simulink model "photorealisticSimulationEngi"  (R2021b)
settings: Solver=FixedStepAuto  StartTime=0.0  StopTime=50  RelTol=1e-3  EnableMultiTasking=on
undefined symbols (not defined in the file): Earth, initialConditions, Lidar, lidarAngles, UAV, UAVSampleTime, uavScenarioBlock, WGS84
libraries: uavsimlib x5, robotcorelib x3, simulink x3, uavutilslib x1, mspfiltlib x1, sim3dcameralib x1, sensorgpslib x1, mspsensorlib x1, aerolibtransform2 x1, sim3dphyssensorlib x1, sim3dlib x1, uavsim3dlib x1
settings Model: DataDictionary=uavPackageDeliveryDataDict.sldd  ModifiedByFormat=The MathWorks, Inc.  Creator=The MathWorks, Inc.  LastModifiedBy=The MathWorks, Inc.
settings SolverCC: AlgebraicLoopSolver=TrustRegion  AutoInsertRateTranBlk=on
settings DataIOCC: LimitDataPoints=on  SaveOutput=off  SaveTime=off  ReturnWorkspaceOutputs=off
settings OptimizationCC: EnhancedBackFolding=on  PassReuseOutputArgsThreshold=0  ZeroExternalMemoryAtStartup=off  ZeroInternalMemoryAtStartup=off  MaxStackSize=64  OptimizeBlockOrder=speed  DifferentSizesBufferReuse=on  OptimizationCustomize=off
settings DebuggingCC: ParameterPrecisionLossMsg=none  ParameterTunabilityLossMsg=error  AllowSymbolicDim=off  SFUnexpectedBacktrackingDiag=warning  SFNoUnconditionalDefaultTransitionDiag=warning  SFExecutionAtInitializationDiag=none  SFMachineParentedDataDiag=warning  ArithmeticOperatorsInVariantConditions=warning
settings HardwareCC: ProdBitPerPointer=32  ProdBitPerSizeT=32  ProdBitPerPtrDiffT=32  ProdLargestAtomicFloat=None  ProdIntDivRoundTo=Undefined  ProdEndianess=Unspecified  ProdWordSize=32  ProdHWDeviceType=Generic->Unspecified (assume 32-bit Generic)
settings ModelReferenceCC: ModelReferenceNumInstancesAllowed=Single  PropagateSignalLabelsOutOfModel=off
settings SFSimCC: SimUseLocalCustomCode=off  MATLABDynamicMemAlloc=off  CustomCodeUndefinedFunction=UseInterfaceOnly  SimTargetLang=C++
settings RTWCC: GenerateReport=on  RTWUseLocalCustomCode=off  LaunchReport=on  TargetLang=C++
settings CodeAppCC: ForceParamTrailComments=on  OperatorAnnotations=on
settings GRTTargetCC: TargetLangStandard=C89/C90 (ANSI)  CodeInterfacePackaging=C++ class
settings ConfigComp: CovMetricSettings=dw  CovSaveCumulativeToWorkspaceVar=on  CovSaveSingleToWorkspaceVar=on  CovExternalEMLEnable=off

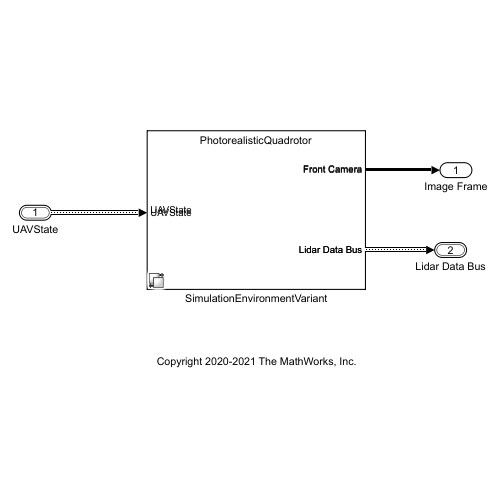
[thumbnail: Simulink's stored preview of the top-level diagram]
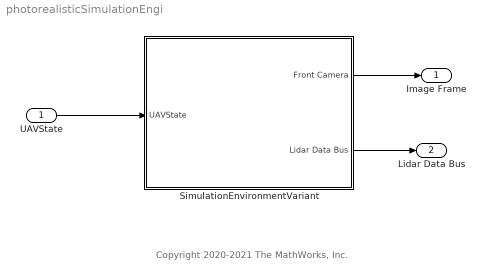
== system photorealisticSimulationEngi ==
  note: Copyright 2020-2021 The MathWorks, Inc.
  UAVState : Inport  OutDataTypeStr=Bus: uavStateBus  BusOutputAsStruct=on
  SimulationEnvironmentVariant : Subsystem  Variant=on  PropagateVariantConditions=on
  Image Frame : Outport
  Lidar Data Bus : Outport  Port=2  OutDataTypeStr=Bus: LidarData
  wires:
  UAVState/1 -> SimulationEnvironmentVariant/1(UAVState)
  SimulationEnvironmentVariant/1(Front Camera) -> Image Frame/1
  SimulationEnvironmentVariant/2(Lidar Data Bus) -> Lidar Data Bus/1

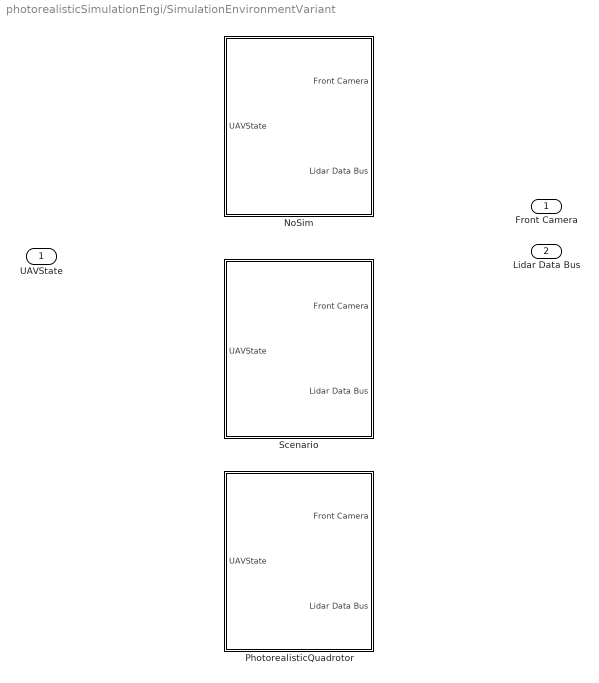
== system photorealisticSimulationEngi/SimulationEnvironmentVariant ==
  UAVState : Inport  OutDataTypeStr=Bus: uavStateBus  PortDimensions=[1 1]  BusOutputAsStruct=on
  NoSim : Subsystem  VariantControl=isPhotoRealisticSim==0
  PhotorealisticQuadrotor : Subsystem  VariantControl=isPhotoRealisticSim==2
  Scenario : Subsystem  VariantControl=isPhotoRealisticSim==1
  Front Camera : Outport  PortDimensions=[ 480 752 3]
  Lidar Data Bus : Outport  Port=2

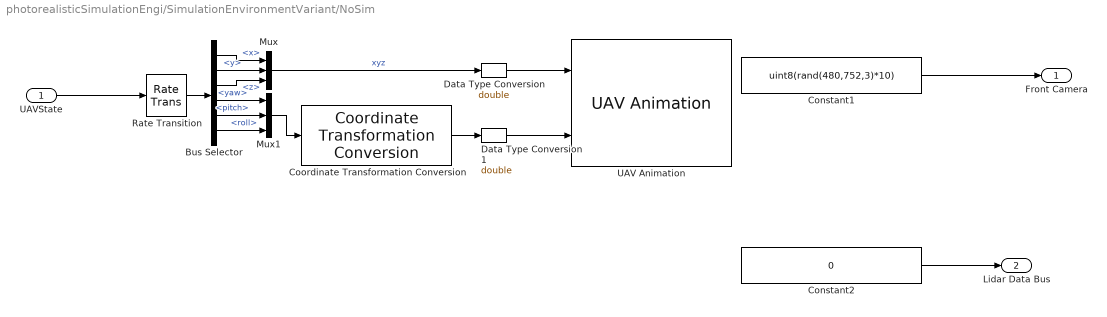
== system photorealisticSimulationEngi/SimulationEnvironmentVariant/NoSim ==
  UAVState : Inport  OutDataTypeStr=Bus: uavStateBus  PortDimensions=[1 1]  SampleTime=UAVSampleTime  BusOutputAsStruct=on
  Bus Selector : BusSelector  OutputSignals=pos_vel.x,pos_vel.y,pos_vel.z,attitude.yaw,attitude.pitch,attitude.roll
  Constant1 : Constant  Value=uint8(rand(480,752,3)*10)
  Constant2 : Constant  Value=0  OutDataTypeStr=Bus: LidarData
  Coordinate Transformation Conversion : robotcorelib/Coordinate Transformation Conversion  InputRepresentation=Euler Angles  InputEulerSequence=ZYX  ShowTrVecInputPort=on  OutputRepresentation=Quaternion  OutputEulerSequence=ZYX  ShowTrVecOutputPort=on  SimulateUsing=Code generation
  Data Type Conversion : DataTypeConversion  OutDataTypeStr=double
  Data Type Conversion1 : DataTypeConversion  OutDataTypeStr=double
  Mux : Mux  Inputs=3
  Mux1 : Mux  Inputs=3
  Rate Transition : RateTransition  OutPortSampleTime=UAVSampleTime*200
  UAV Animation : uavutilslib/UAV Animation  UAVType=Multirotor  UAVSize=1  InertialZDirection=Down  SampleTime=UAVSampleTime*200
      settings: SourceProductName=UAV Toolbox
  Front Camera : Outport  OutDataTypeStr=uint8  PortDimensions=[480 752 3]
  Lidar Data Bus : Outport  Port=2
  wires:
  Constant1/1 -> Front Camera/1
  Constant2/1 -> Lidar Data Bus/1
  Bus Selector/1 -> Mux/1  "<x>"
  Bus Selector/2 -> Mux/2  "<y>"
  Bus Selector/3 -> Mux/3  "<z>"
  Mux/1 -> Data Type Conversion/1  "xyz"
  Bus Selector/6 -> Mux1/3  "<roll>"
  Bus Selector/5 -> Mux1/2  "<pitch>"
  Bus Selector/4 -> Mux1/1  "<yaw>"
  Coordinate Transformation Conversion/1 -> Data Type Conversion1/1
  Mux1/1 -> Coordinate Transformation Conversion/1
  Data Type Conversion1/1 -> UAV Animation/2
  UAVState/1 -> Rate Transition/1
  Data Type Conversion/1 -> UAV Animation/1
  Rate Transition/1 -> Bus Selector/1

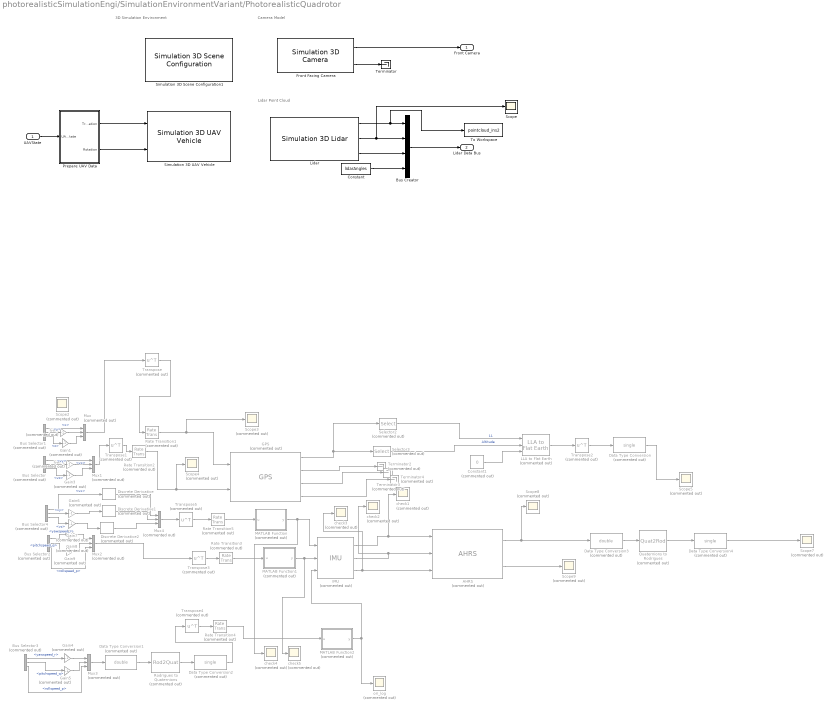
== system photorealisticSimulationEngi/SimulationEnvironmentVariant/PhotorealisticQuadrotor ==
  note: 3D Simulation Environment
  note: Camera Model
  note: Lidar Point Cloud
  UAVState : Inport  PortDimensions=[1 1]  SampleTime=[0.01,0]  BusOutputAsStruct=on
  AHRS : mspfiltlib/AHRS  Commented=on  DispRefFrame=NED  DecimationFactor=1  InitialProcessNoise=ahrsfilter.defaultProcessNoise  OrientationFormat=quaternion  SimulateUsing=Interpreted execution  AccelerometerNoise=0.0001924722  GyroscopeNoise=9.1385e-5  MagnetometerNoise=0.1  GyroscopeDriftNoise=3.0462e-13  LinearAccelerationNoise=0.0096236100000000012  MagneticDisturbanceNoise=0.5  LinearAccelerationDecayFactor=0.5  MagneticDisturbanceDecayFactor=0.5  ExpectedMagneticFieldStrength=50
      settings: SourceProductBaseCode=TF,NV
  Bus Creator : BusCreator  Inputs=4  OutDataTypeStr=Bus: LidarData  NonVirtualBus=on
      settings: InheritFromInputs=off
  Bus Selector : BusSelector  Commented=on  OutputSignals=pos_vel.vx,pos_vel.vy,pos_vel.vz
  Bus Selector1 : BusSelector  Commented=on  OutputSignals=pos_vel.x,pos_vel.y,pos_vel.z
  Bus Selector2 : BusSelector  Commented=on  OutputSignals=attitude.yawspeed_r,attitude.pitchspeed_q,attitude.rollspeed_p
  Bus Selector3 : BusSelector  Commented=on  OutputSignals=attitude.yawspeed_r,attitude.pitchspeed_q,attitude.rollspeed_p
  Bus Selector4 : BusSelector  Commented=on  OutputSignals=pos_vel.vx,pos_vel.vy,pos_vel.vz
  Constant : Constant  Value=lidarAngles
  Constant1 : Constant  Commented=on  Value=0
  Data Type Conversion : DataTypeConversion  Commented=on  OutDataTypeStr=single
  Data Type Conversion1 : DataTypeConversion  Commented=on  OutDataTypeStr=double
  Data Type Conversion2 : DataTypeConversion  Commented=on  OutDataTypeStr=single
  Data Type Conversion3 : DataTypeConversion  Commented=on  OutDataTypeStr=double
  Data Type Conversion4 : DataTypeConversion  Commented=on  OutDataTypeStr=single
  Discrete Derivative : simulink/Discrete/Discrete Derivative  Commented=on  gainval=1.0  ICPrevScaledInput=0.0  OutMin=[]  OutMax=[]  OutDataType=fixdt(1, 16)  OutScaling=2^-10  DoSatur=off
  Discrete Derivative1 : simulink/Discrete/Discrete Derivative  Commented=on  gainval=1.0  ICPrevScaledInput=0.0  OutMin=[]  OutMax=[]  OutDataType=fixdt(1, 16)  OutScaling=2^-10  DoSatur=off
  Discrete Derivative2 : simulink/Discrete/Discrete Derivative  Commented=on  gainval=1.0  ICPrevScaledInput=0.0  OutMin=[]  OutMax=[]  OutDataType=fixdt(1, 16)  OutScaling=2^-10  DoSatur=off
  Front Facing Camera : sim3dcameralib/Simulation 3D Camera  Priority=1  sensorTag=Sim3dSensor2  sensorId=2  sensorName=Sim3dSensor2  vehTagList={'Scene Origin';'SimulinkVehicle1'}  vehTag=SimulinkVehicle1  mountLoc=Origin  offsetFlag=on  tmountOffset=[0 0 -0.15]  extTmount=off  rmountOffset=[0, 0, 0]  extRmount=off  FocalLength=[1109, 1109]  OpticalCenter=[376, 240]  ImageSize=[480, 752]  RadialDistortion=[0, 0]  TangentialDistortion=[0, 0]  SensorSkew=0  DepthOutportEnabled=on  SemanticOutportEnabled=off  TransformOutportEnabled=off  SampleTime=UAVSampleTime*20  mountPoint=[0 0 -0.15]  mountOrientation=[0 0 0]  aMode=4  ID=2
      settings: SourceProductBaseCode=AE,DR,UV,VE
  GPS : sensorgpslib/GPS  Commented=on  DispRefFrame=NED  PositionInputFormat=Local  ReferenceLocation=[41.8856528 -87.6556726 0]  HorizontalPositionAccuracy=1.6  VerticalPositionAccuracy=3  VelocityAccuracy=0.1  DecayFactor=0.999  SeedDouble=67  SimulateUsing=Interpreted execution
      settings: SourceProductBaseCode=TF,NV,UV
  Gain{,1..9} (10 alike) : Gain  Commented=on  Gain=-1
  IMU : mspsensorlib/IMU  Commented=on  DispRefFrame=NED  Temperature=25  MagneticFieldNED=[ 27.5550, -2.4169, -16.0849 ]  MagneticFieldENU=[ -2.4169, 27.5550, 16.0849 ]  SeedDouble=67  SimulateUsing=Interpreted execution  AccelParamsMeasurementRange=Inf  AccelParamsResolution=0  AccelParamsConstantBias=[ 0, 0, 0 ]  AccelParamsAxesMisalignment=[ 100, 0, 0; 0, 100, 0; 0, 0, 100 ]  AccelParamsNoiseDensity=[ 0, 0, 0 ]  AccelParamsBiasInstability=[ 0, 0, 0 ]  AccelParamsRandomWalk=[ 0, 0, 0 ]  AccelParamsTemperatureBias=[ 0, 0, 0 ]  AccelParamsTemperatureScaleFactor=[ 0, 0, 0 ]  GyroParamsMeasurementRange=Inf  GyroParamsResolution=0  GyroParamsConstantBias=[ 0, 0, 0 ]  GyroParamsAxesMisalignment=[ 100, 0, 0; 0, 100, 0; 0, 0, 100 ]  GyroParamsAccelerationBias=[ 0, 0, 0 ]  GyroParamsNoiseDensity=[ 0, 0, 0 ]  GyroParamsBiasInstability=[ 0, 0, 0 ]  GyroParamsRandomWalk=[ 0, 0, 0 ]  GyroParamsTemperatureBias=[ 0, 0, 0 ]  GyroParamsTemperatureScaleFactor=[ 0, 0, 0 ]  MagParamsMeasurementRange=Inf  MagParamsResolution=0  MagParamsConstantBias=[ 0, 0, 0 ]  MagParamsAxesMisalignment=[ 100, 0, 0; 0, 100, 0; 0, 0, 100 ]  MagParamsNoiseDensity=[ 0, 0, 0 ]  MagParamsBiasInstability=[ 0, 0, 0 ]  MagParamsRandomWalk=[ 0, 0, 0 ]  MagParamsTemperatureBias=[ 0, 0, 0 ]  MagParamsTemperatureScaleFactor=[ 0, 0, 0 ]
      settings: SourceProductBaseCode=TF,NV
  LLA to Flat Earth : aerolibtransform2/LLA to Flat Earth  Commented=on  units=Metric (MKS)  ptype=Earth (WGS84)  F=1/298.257223563  R=6378137  refPosPort=off  LL0=[41.8856528 -87.6556726]  psi=0
      settings: SourceProductBaseCode=AE
  Lidar : sim3dphyssensorlib/Simulation 3D Lidar  Priority=1  sensorTag=Sim3dSensor3  sensorId=3  sensorName=Sim3dSensor3  vehTagList={'Scene Origin';'SimulinkVehicle1'}  vehTag=SimulinkVehicle1  mountLoc=Origin  offsetFlag=on  tmountOffset=[0, 0, 0.35]  rmountOffset=[0, 0, 0]  DetectionRange=90  RangeResolution=0.002  VerticalFOV=40  VerticalResolution=1.25  HorizontalFOV=360  HorizontalResolution=0.332409972299169  DistanceOutportEnabled=off  TransformOutportEnabled=on  SampleTime=UAVSampleTime*100  mountPoint=[0 0 0.35]  mountOrientation=[0 0 0]  aMode=4  ID=3
      settings: SourceProductBaseCode=AE,DR,UV,VE
  MATLAB Function : MATLAB Function  Commented=on  TreatAsAtomicUnit=on
  MATLAB Function1 : MATLAB Function  Commented=on  TreatAsAtomicUnit=on
  MATLAB Function2 : MATLAB Function  Commented=on  TreatAsAtomicUnit=on
  Mux{,1..4} (5 alike) : Mux  Commented=on  Inputs=3
  Prepare UAV Data : Subsystem
  Quaternions to Rodrigues : Quat2Rod  Commented=on
  Rate Transition{1..5} (5 alike) : RateTransition  Commented=on  OutPortSampleTime=0.5
  Rodrigues to Quaternions : Rod2Quat  Commented=on
  Scope : Scope
  Scope{2..5,7..9} (7 alike) : Scope  Commented=on
  Selector2 : Selector  Commented=on  InputPortWidth=3  IndexOptions=Index vector (dialog)  Indices=[1 2]  OutputSizes=1
  Selector3 : Selector  Commented=on  InputPortWidth=3  IndexOptions=Index vector (dialog)  Indices=[3]  OutputSizes=1
  Simulation 3D Scene Configuration1 : sim3dlib/Simulation 3D Scene Configuration  Priority=0  ProjectFormat_internal=Default Scenes  ProjectFormat=Default Scenes  SceneDesc=US city block  ProjectName=D:\Program Files\MATLAB\R2021b\toolbox\shared\sim3d_projects\automotive_project\UE4\WindowsNoEditor\VehicleSimulation.exe  ScenePath=/Game/Maps/HwStrght  vehTagList={'Scene Origin';'SimulinkVehicle1'}  vehTag=SimulinkVehicle1  OpVisEn=off  Ts=0.1  EnableWindow=on  EnableWeather=off  SunAltitude=40.0  SunAzimuth=90  clouds=10  wind=1  fog=0  rain=0  sensorTag=MainCamera5  sensorId=5  sensorName=MainCamera5  mountLoc=Origin  offsetFlag=off  tmountOffset=[0, 0, 0]  rmountOffset=[0, 0, 0]  HorizontalResolution=1280  VerticalResolution=720  HorizontalFOV=60  mountPoint=[0 0 0]  mountOrientation=[0 0 0]  aMode=4  ID=5
      settings: SourceProductBaseCode=AE,DR,UV,VE
  Simulation 3D UAV Vehicle : uavsim3dlib/Simulation 3D UAV Vehicle  Priority=-1  Mesh=Quadrotor  MeshPath=/MathWorksUAVContent/UAVs/HexaRotorUAV/HexaRotor.HexaRotor  Color=Blue  ActorName=SimulinkVehicle1  InitialTranslation=[-186 105 0]  InitialRotation=[0 0 0]  SampleTime=-1  ActorType=SimulinkVehicle  ID=1  aMode=4  ActorTag=SimulinkVehicle1
      settings: SourceProductBaseCode=UV
  Terminator : Terminator
  Terminator2 : Terminator  Commented=on
  Terminator3 : Terminator  Commented=on
  Terminator4 : Terminator  Commented=on
  To Workspace : ToWorkspace  VariableName=pointcloud_ins2  SaveFormat=Timeseries  SampleTime=-1
  Transpose{,1..5} (6 alike) : Math  Commented=on  Operator=transpose  SaturateOnIntegerOverflow=on
  check{1..5} (5 alike) : Scope  Commented=on
  ori_log : Scope  Commented=on
  Front Camera : Outport  PortDimensions=[ 480 752 3]
  Lidar Data Bus : Outport  Port=2
  wires:
  Front Facing Camera/1 -> Front Camera/1
  Lidar/1 -> To Workspace/1, Bus Creator/1
  Lidar/2 -> Bus Creator/2, Scope/1
  Bus Creator/1 -> Lidar Data Bus/1
  UAVState/1 -> Prepare UAV Data/1(UAVState)
  Front Facing Camera/2 -> Terminator/1
  Prepare UAV Data/1(Translation) -> Simulation 3D UAV Vehicle/1
  Prepare UAV Data/2(Rotation) -> Simulation 3D UAV Vehicle/2
  Constant/1 -> Bus Creator/4
  Bus Selector1/1 -> Mux/1  "<x>"
  Bus Selector/1 -> Mux1/1  "<vx>"
  Lidar/3 -> Bus Creator/3
  Bus Selector1/2 -> Gain/1  "<y>"
  Gain/1 -> Mux/2
  Bus Selector1/3 -> Gain1/1  "<z>"
  Gain1/1 -> Mux/3
  Rate Transition1/1 -> Scope3/1, GPS/1
  Rate Transition2/1 -> Scope4/1, GPS/2
  Gain2/1 -> Mux1/2
  Bus Selector/2 -> Gain2/1  "<vy>"
  Bus Selector/3 -> Gain3/1  "<vz>"
  Gain3/1 -> Mux1/3
  GPS/2 -> Terminator2/1
  GPS/3 -> Terminator3/1
  GPS/4 -> Terminator4/1
  Mux/1 -> Transpose/1
  Transpose/1 -> Rate Transition1/1
  Mux1/1 -> Transpose1/1
  Transpose1/1 -> Rate Transition2/1
  Constant1/1 -> LLA to Flat Earth/3
  GPS/1 -> Selector3/1, Selector2/1
  Selector2/1 -> LLA to Flat Earth/1  "LL"
  Selector3/1 -> LLA to Flat Earth/2  "Altitude"
  LLA to Flat Earth/1 -> Transpose2/1
  Transpose2/1 -> Data Type Conversion/1
  Data Type Conversion/1 -> Scope5/1
  Transpose3/1 -> Rate Transition3/1
  Transpose4/1 -> Rate Transition4/1
  Rate Transition4/1 -> MATLAB Function2/1(u)
  Bus Selector4/2 -> Gain6/1  "<vy>"
  Bus Selector4/3 -> Gain7/1  "<vz>"
  Bus Selector4/1 -> Discrete Derivative/1  "<vx>"
  Discrete Derivative/1 -> Mux4/1
  Gain6/1 -> Discrete Derivative1/1
  Discrete Derivative1/1 -> Mux4/2
  Gain7/1 -> Discrete Derivative2/1
  Discrete Derivative2/1 -> Mux4/3
  Transpose5/1 -> Rate Transition5/1
  Mux3/1 -> Data Type Conversion1/1
  Data Type Conversion1/1 -> Rodrigues to Quaternions/1
  Rodrigues to Quaternions/1 -> Data Type Conversion2/1
  IMU/1 -> check1/1, AHRS/1
  IMU/2 -> check2/1, AHRS/2
  IMU/3 -> check3/1, AHRS/3
  AHRS/2 -> Scope9/1
  Data Type Conversion3/1 -> Quaternions to Rodrigues/1
  Quaternions to Rodrigues/1 -> Data Type Conversion4/1
  Data Type Conversion4/1 -> Scope7/1
  AHRS/1 -> Data Type Conversion3/1, Scope8/1
  Bus Selector2/3 -> Mux2/3  "<rollspeed_p>"
  Bus Selector2/1 -> Gain8/1  "<yawspeed_r>"
  Gain8/1 -> Mux2/1
  Bus Selector2/2 -> Gain9/1  "<pitchspeed_q>"
  Gain9/1 -> Mux2/2
  Bus Selector3/1 -> Gain4/1  "<yawspeed_r>"
  Gain4/1 -> Mux3/1
  Bus Selector3/2 -> Gain5/1  "<pitchspeed_q>"
  Gain5/1 -> Mux3/2
  Bus Selector3/3 -> Mux3/3  "<rollspeed_p>"
  Mux4/1 -> Transpose5/1
  Mux2/1 -> Transpose3/1
  Data Type Conversion2/1 -> Transpose4/1
  MATLAB Function/1(y) -> check4/1, IMU/1
  Rate Transition5/1 -> MATLAB Function/1(u)
  Rate Transition3/1 -> MATLAB Function1/1(u)
  MATLAB Function1/1(y) -> check5/1, IMU/2
  MATLAB Function2/1(y) -> IMU/3, ori_log/1

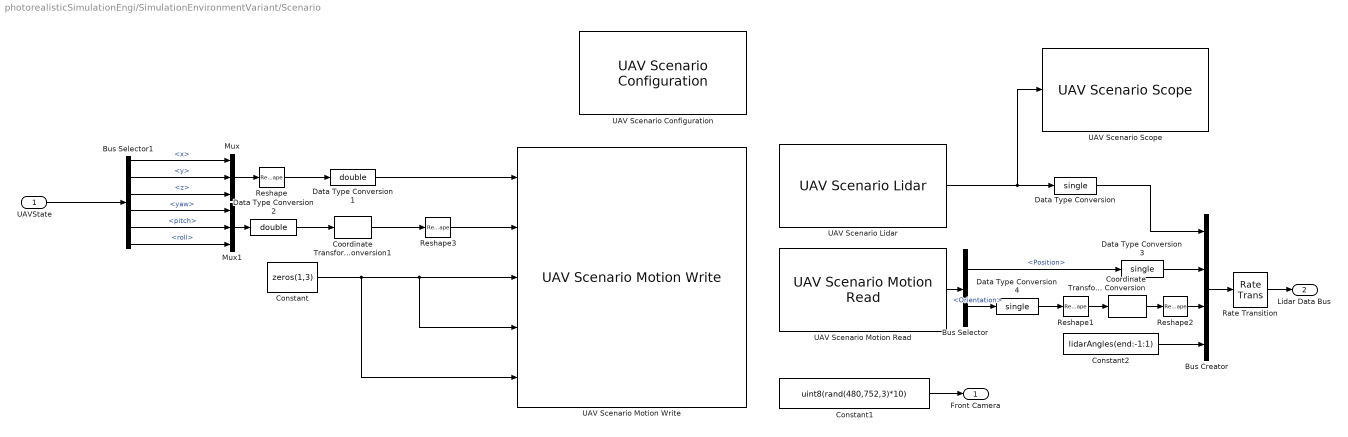
== system photorealisticSimulationEngi/SimulationEnvironmentVariant/Scenario ==
  UAVState : Inport
  Bus Creator : BusCreator  Inputs=4  OutDataTypeStr=Bus: LidarData  NonVirtualBus=on
      settings: InheritFromInputs=off
  Bus Selector : BusSelector  OutputSignals=Position,Orientation
  Bus Selector1 : BusSelector  OutputSignals=pos_vel.x,pos_vel.y,pos_vel.z,attitude.yaw,attitude.pitch,attitude.roll
  Constant : Constant  Value=zeros(1,3)
  Constant1 : Constant  Value=uint8(rand(480,752,3)*10)
  Constant2 : Constant  Value=lidarAngles(end:-1:1)
  Coordinate Transformation Conversion : robotcorelib/Coordinate Transformation Conversion  InputRepresentation=Quaternion  InputEulerSequence=ZYX  ShowTrVecInputPort=on  OutputRepresentation=Euler Angles  OutputEulerSequence=ZYX  ShowTrVecOutputPort=on  SimulateUsing=Code generation
      settings: SourceProductBaseCode=NV,RO,RR,UV
  Coordinate Transformation Conversion1 : robotcorelib/Coordinate Transformation Conversion  InputRepresentation=Euler Angles  InputEulerSequence=ZYX  ShowTrVecInputPort=on  OutputRepresentation=Quaternion  OutputEulerSequence=ZYX  ShowTrVecOutputPort=on  SimulateUsing=Code generation
      settings: SourceProductBaseCode=NV,RO,RR,UV
  Data Type Conversion : DataTypeConversion  OutDataTypeStr=single
  Data Type Conversion1 : DataTypeConversion  OutDataTypeStr=double
  Data Type Conversion2 : DataTypeConversion  OutDataTypeStr=double
  Data Type Conversion3 : DataTypeConversion  OutDataTypeStr=single
  Data Type Conversion4 : DataTypeConversion  OutDataTypeStr=single
  Mux : Mux  Inputs=3
  Mux1 : Mux  Inputs=3
  Rate Transition : RateTransition  OutPortSampleTime=0.5
  Reshape : Reshape  OutputDimensionality=Row vector (2-D)
  Reshape1 : Reshape  OutputDimensionality=Column vector (2-D)
  Reshape2 : Reshape  OutputDimensionality=Row vector (2-D)
  Reshape3 : Reshape  OutputDimensionality=Row vector (2-D)
  UAV Scenario Configuration : uavsimlib/UAV Scenario Configuration  Priority=-1  UAVScenarioObject=uavScenarioBlock(initialConditions.posNED, [0 0 0])  SampleTime=0.5  UpdateParam=true  SensorMotionBusName='SensorMotionBus'  PlatformMotionBusName='PlatformMotionBus'  ScenarioMotionBusName='ScenarioMotionBus'  ScenarioMotionSignalName='ScenarioMotions'
      settings: SourceProductBaseCode=UV
  UAV Scenario Lidar : uavsimlib/UAV Scenario Lidar  Priority=1  SensorName=UAV/Lidar  MaxRange=90  RangeAccuracy=0.002  AzimuthLimits=[ -180, 180 ]  AzimuthResolution=0.3324099  ElevationLimits=[ -20, 20 ]  ElevationResolution=1.25  HasNoise=on  HasOrganizedOutput=on  SampleTime=0.5
      settings: SourceProductBaseCode=UV
  UAV Scenario Motion Read : uavsimlib/UAV Scenario Motion Read  Priority=1  EntityName='UAV/Lidar'  ReferenceFrame=NED
      settings: SourceProductBaseCode=UV
  UAV Scenario Motion Write : uavsimlib/UAV Scenario Motion Write  Priority=0  PlatName='UAV'  ReferenceFrame=NED
      settings: SourceProductBaseCode=UV
  UAV Scenario Scope : uavsimlib/UAV Scenario Scope  Priority=1  SensorNameTable={'UAV/Lidar', 'on'}  SampleTime=0.5
      settings: SourceProductBaseCode=UV
  Front Camera : Outport
  Lidar Data Bus : Outport  Port=2
  wires:
  Bus Selector1/5 -> Mux1/2  "<pitch>"
  Bus Selector1/4 -> Mux1/1  "<yaw>"
  Reshape3/1 -> UAV Scenario Motion Write/2
  Data Type Conversion3/1 -> Bus Creator/2
  Coordinate Transformation Conversion1/1 -> Reshape3/1
  Coordinate Transformation Conversion/1 -> Reshape2/1
  UAV Scenario Motion Read/1 -> Bus Selector/1
  Bus Selector1/2 -> Mux/2  "<y>"
  Bus Selector/1 -> Data Type Conversion3/1  "<Position>"
  Bus Selector/2 -> Data Type Conversion4/1  "<Orientation>"
  Data Type Conversion1/1 -> UAV Scenario Motion Write/1
  Rate Transition/1 -> Lidar Data Bus/1
  Bus Selector1/6 -> Mux1/3  "<roll>"
  Data Type Conversion4/1 -> Reshape1/1
  Reshape/1 -> Data Type Conversion1/1
  Mux/1 -> Reshape/1
  Constant1/1 -> Front Camera/1
  Data Type Conversion/1 -> Bus Creator/1
  Bus Selector1/3 -> Mux/3  "<z>"
  UAVState/1 -> Bus Selector1/1
  UAV Scenario Lidar/1 -> UAV Scenario Scope/1, Data Type Conversion/1
  Bus Creator/1 -> Rate Transition/1
  Constant/1 -> UAV Scenario Motion Write/5, UAV Scenario Motion Write/4, UAV Scenario Motion Write/3
  Reshape2/1 -> Bus Creator/3
  Data Type Conversion2/1 -> Coordinate Transformation Conversion1/1
  Reshape1/1 -> Coordinate Transformation Conversion/1
  Mux1/1 -> Data Type Conversion2/1
  Bus Selector1/1 -> Mux/1  "<x>"
  Constant2/1 -> Bus Creator/4

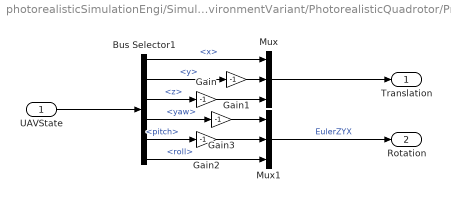
== system photorealisticSimulationEngi/SimulationEnvironmentVariant/PhotorealisticQuadrotor/Prepare UAV Data ==
  UAVState : Inport
  Bus Selector1 : BusSelector  OutputSignals=pos_vel.x,pos_vel.y,pos_vel.z,attitude.yaw,attitude.pitch,attitude.roll
  Gain{,1..3} (4 alike) : Gain  Gain=-1
  Mux : Mux  Inputs=3
  Mux1 : Mux  Inputs=3
  Translation : Outport
  Rotation : Outport  Port=2
  wires:
  UAVState/1 -> Bus Selector1/1
  Mux/1 -> Translation/1
  Mux1/1 -> Rotation/1  "EulerZYX"
  Bus Selector1/4 -> Gain3/1  "<yaw>"
  Bus Selector1/5 -> Gain2/1  "<pitch>"
  Bus Selector1/6 -> Mux1/3  "<roll>"
  Bus Selector1/3 -> Gain/1  "<z>"
  Bus Selector1/2 -> Gain1/1  "<y>"
  Bus Selector1/1 -> Mux/1  "<x>"
  Gain/1 -> Mux/3
  Gain1/1 -> Mux/2
  Gain2/1 -> Mux1/2
  Gain3/1 -> Mux1/1

== matlab function photorealisticSimulationEngi/SimulationEnvironmentVariant/PhotorealisticQuadrotor/MATLAB Function ==
  data: u input; y output
function y = add_bias(u)

if u(1) == 0 && u(2) == 0 && u(3) == 0
    u = u + [0.01 0.01 0.01];
end
y = u;

== matlab function photorealisticSimulationEngi/SimulationEnvironmentVariant/PhotorealisticQuadrotor/MATLAB Function2 ==
  data: u input; y output
function y = add_bias2(u)

if u(1) == 0 && u(2) == 0 && u(3) == 0 && u(4) == 0
    u = u + [0.01 0.01 0.01 0.01];
end
y = u;

== matlab function photorealisticSimulationEngi/SimulationEnvironmentVariant/PhotorealisticQuadrotor/MATLAB Function1 ==
  data: u input; y output
function y = add_bias(u)

if u(1) == 0 && u(2) == 0 && u(3) == 0
    u = u + [0.01 0.01 0.01];
end
y = u;
